simulink model "ad9361_rx_wlan_testbench_targeting_org"  (Simulink 10.0)
settings: Solver=FixedStepDiscrete  StartTime=0.0  StopTime=2  RelTol=1e-3
InitFcn:
  | % General
  | FFT = 64;
  | LSTFSymbol = FFT/4;
  | FS = 20e6;
  | 
  | % NCO
  | Fs = 20e6;
  | res = 0.05;
  | SFDR = 100;
  | N = ceil(log2(Fs/res));
  | %trueRes = Fs/(2^N);
  | %phaseInc = round(Fc*2^N/Fs);
  | QAB = round((SFDR-12)/6);
  | Dither = N - QAB;
  | 
  | %% LLTF
  | a = load('lltf.mat');
  | lltfFlip = conj(flipud(a.LLTF(:, 1)));
  | 
  | lltfFlip = lltfFlip./(max(abs(lltfFlip))) .* 2^0;
libraries: simulink x9, dsphdlfiltering x5, hdlsllib x4, commsource2 x1, dspmathops x1, dspsigops x1
(part 2 of 2)

== system ad9361_rx_wlan_testbench_targeting_org/HDL_DUT/ReceiverDSP/SymbolTiming/Symbol Timing Validate/PeakCheck ==
  symSync : Inport
  AND : Logic  IconShape=distinctive  AllPortsSameDT=off  OutDataTypeStr=boolean
  Delay7 : Delay  DelayLength=1
  Delay8 : Delay
  GreaterThan1 : RelationalOperator  Operator=>  OutDataTypeStr=boolean  RndMeth=Simplest
  GreaterThan2 : RelationalOperator  Operator=>  OutDataTypeStr=boolean  RndMeth=Simplest
  Out1 : Outport  VectorParamsAs1DForOutWhenUnconnected=off
  wires:
  GreaterThan1/1 -> AND/2
  GreaterThan2/1 -> AND/1
  symSync/1 -> Delay8/1, Delay7/1, GreaterThan2/2
  Delay7/1 -> GreaterThan2/1, GreaterThan1/1
  Delay8/1 -> GreaterThan1/2
  AND/1 -> Out1/1

== matlab function CheckPayloadEnable/Check LSIG1 ==
  data: start input double; data input double; valid output double; goodPackets output double; badPackets output double
function [valid,goodPackets,badPackets] = fcn(start,data)
%#codegen
% coder.extrinsic('offline');

persistent buff counter cfgRec largerCount chanEst noiseVar cfgNonHT numDataSym
persistent goodPacketsCount badPacketsCount
N = 160+80; 
M = 1e6;

if isempty(buff)
    buff = complex(zeros(M,1));
    counter = int16(N+1);
    cfgRec = wlanRecoveryConfig('EqualizationMethod', 'ZF');
    largerCount = 0;
    cfgNonHT = wlanNonHTConfig;
    numDataSym = 0;
    chanEst = 0;
    noiseVar = 0;
    goodPacketsCount = 0;
    badPacketsCount = 0;
end

valid = false;

if start
    counter = int16(1);
elseif counter <= N
    counter = counter + int16(1);
end

if counter<N
    buff(counter) = data;
end

if counter == N
    counter = N + int16(1);
    rxLLTF = buff(1:160);
    rxLSIG = buff(161:160+80);
    chanBW = 'CBW20';
    % Perform channel estimation based on L-LTF
    demodLLTF = wlanLLTFDemodulate(rxLLTF, chanBW, 1);
    noiseVar = helperNoiseEstimate(demodLLTF);
    chanEst = wlanLLTFChannelEstimate(demodLLTF, chanBW);
    % Recover information bits in L-SIG
    [recLSIGBits,failParityCheck] = wlanLSIGRecover(rxLSIG, chanEst, noiseVar, chanBW);
    if ~failParityCheck %isequal(ref,recLSIGBits.')
        rate = bi2de(double(recLSIGBits(1:3).'), 'left-msb');
        if rate <= 1
            cfgNonHT.MCS = rate + 6;
        else
            cfgNonHT.MCS = mod(rate, 6);
        end
        fprintf('LSIG GOOD\n');
        cfgNonHT.PSDULength = bi2de(double(recLSIGBits(6:17)'));
        largerCount = 1;
        numDataSym = offline(cfgNonHT);
    else
        fprintf('LSIG Invalid\n');
        badPacketsCount = badPacketsCount + 1;
    end
end

if largerCount > 0
    buff(largerCount) = data;
    largerCount = largerCount + 1;
    if largerCount > 80*numDataSym
        % Recover payload bits
        recBits = wlanNonHTDataRecover(buff(2:80*numDataSym+1), chanEst, ...
            noiseVar, cfgNonHT, cfgRec);        
        % Evaluate recovered bits
        [validBeacon, MPDU] = nonHTBeaconRxMPDUDecode(recBits);
        if validBeacon
            goodPacketsCount = goodPacketsCount + 1;
            % nonHTBeaconRxOutputDisplay(MPDU); % Display SSID
            fprintf('Good packets captured: %d\n',int16(goodPacketsCount));
        else
            badPacketsCount = badPacketsCount + 1;
            fprintf('Bad packets captured: %d\n',int16(badPacketsCount));
        end
        largerCount = 0;
        valid = true;
    end
end

goodPackets = goodPacketsCount;
badPackets = badPacketsCount;

end

== matlab function CheckPayload/Check LSIG1 ==
  data: start input double; data input double; valid output double; goodPackets output double; badPackets output double
function [valid,goodPackets,badPackets] = fcn(start,data)
%#codegen
% coder.extrinsic('offline');

persistent buff counter cfgRec largerCount chanEst noiseVar cfgNonHT numDataSym
persistent goodPacketsCount badPacketsCount
N = 160+80; 
M = 1e6;

if isempty(buff)
    buff = complex(zeros(M,1));
    counter = int16(N+1);
    cfgRec = wlanRecoveryConfig('EqualizationMethod', 'ZF');
    largerCount = 0;
    cfgNonHT = wlanNonHTConfig;
    numDataSym = 0;
    chanEst = 0;
    noiseVar = 0;
    goodPacketsCount = 0;
    badPacketsCount = 0;
end

valid = false;

if start
    counter = int16(1);
elseif counter <= N
    counter = counter + int16(1);
end

if counter<N
    buff(counter) = data;
end

if counter == N
    counter = N + int16(1);
    rxLLTF = buff(1:160);
    rxLSIG = buff(161:160+80);
    chanBW = 'CBW20';
    % Perform channel estimation based on L-LTF
    demodLLTF = wlanLLTFDemodulate(rxLLTF, chanBW, 1);
    noiseVar = helperNoiseEstimate(demodLLTF);
    chanEst = wlanLLTFChannelEstimate(demodLLTF, chanBW);
    % Recover information bits in L-SIG
    [recLSIGBits,failParityCheck] = wlanLSIGRecover(rxLSIG, chanEst, noiseVar, chanBW);
    if ~failParityCheck %isequal(ref,recLSIGBits.')
        rate = bi2de(double(recLSIGBits(1:3).'), 'left-msb');
        if rate <= 1
            cfgNonHT.MCS = rate + 6;
        else
            cfgNonHT.MCS = mod(rate, 6);
        end
        fprintf('LSIG GOOD\n');
        cfgNonHT.PSDULength = bi2de(double(recLSIGBits(6:17)'));
        largerCount = 1;
        numDataSym = offline(cfgNonHT);
    else
        fprintf('LSIG Invalid\n');
        badPacketsCount = badPacketsCount + 1;
    end
end

if largerCount > 0
    buff(largerCount) = data;
    largerCount = largerCount + 1;
    if largerCount > 80*numDataSym
        % Recover payload bits
        recBits = wlanNonHTDataRecover(buff(2:80*numDataSym+1), chanEst, ...
            noiseVar, cfgNonHT, cfgRec);        
        % Evaluate recovered bits
        [validBeacon, MPDU] = nonHTBeaconRxMPDUDecode(recBits);
        if validBeacon
            goodPacketsCount = goodPacketsCount + 1;
%             nonHTBeaconRxOutputDisplay(MPDU); % Display SSID
            fprintf('Good packets captured: %d\n',int16(goodPacketsCount));
        else
            badPacketsCount = badPacketsCount + 1;
            fprintf('Bad packets captured: %d\n',int16(badPacketsCount));
        end
        largerCount = 0;
        valid = true;
    end
end

goodPackets = goodPacketsCount;
badPackets = badPacketsCount;

end

== matlab function HDL_DUT/Output Interface/Enabled Counter/MATLAB Function ==
  data: enable input double; out output double; maxCount input double
function out = fcn(enable, maxCount)
%#codegen

persistent counter

if isempty(counter)
   counter = uint32(0); 
end

if enable && counter == uint32(0)
    out = true;
    counter = uint32(maxCount-1);
elseif counter > uint32(0)
    out = true;
    counter = counter - uint32(1);
else
    out = false;
end
